simulink model "correlator_core"  (Simulink 7.1)
settings: Solver=ode45  StartTime=0.0  StopTime=10000  RelTol=1e-3
libraries: xbsIndex_r4 x658, cfa_library x168, casper_library_delays x4, casper_library_misc x2
(part 6 of 9)

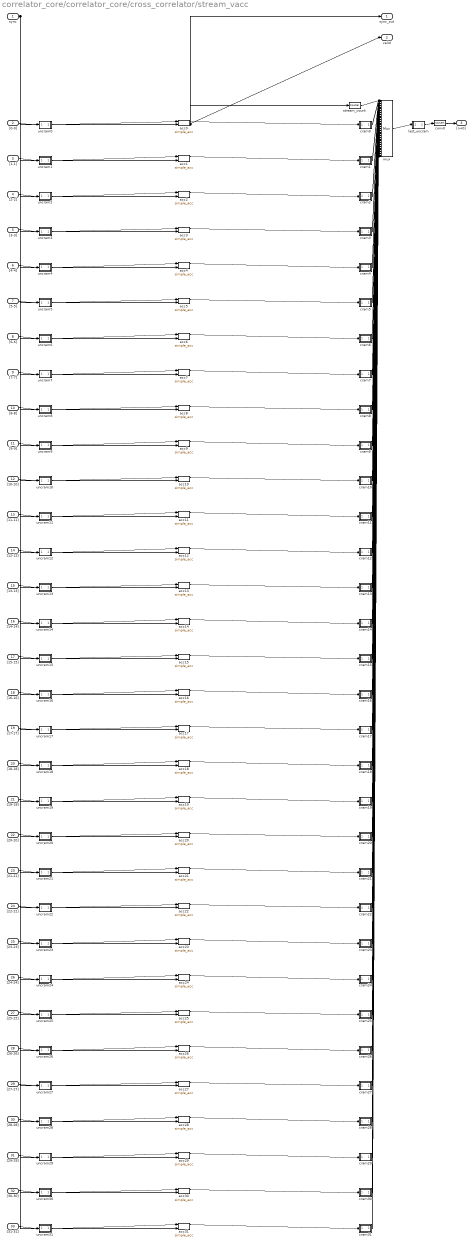
== system correlator_core/correlator_core/cross_correlator/stream_vacc ==
  sync : Inport
  "[0-0]" : Inport  Port=2
  "[1-1]" : Inport  Port=3
  "[2-2]" : Inport  Port=4
  "[3-3]" : Inport  Port=5
  "[4-4]" : Inport  Port=6
  "[5-5]" : Inport  Port=7
  "[6-6]" : Inport  Port=8
  "[7-7]" : Inport  Port=9
  "[8-8]" : Inport  Port=10
  "[9-9]" : Inport  Port=11
  "[10-10]" : Inport  Port=12
  "[11-11]" : Inport  Port=13
  "[12-12]" : Inport  Port=14
  "[13-13]" : Inport  Port=15
  "[14-14]" : Inport  Port=16
  "[15-15]" : Inport  Port=17
  "[16-16]" : Inport  Port=18
  "[17-17]" : Inport  Port=19
  "[18-18]" : Inport  Port=20
  "[19-19]" : Inport  Port=21
  "[20-20]" : Inport  Port=22
  "[21-21]" : Inport  Port=23
  "[22-22]" : Inport  Port=24
  "[23-23]" : Inport  Port=25
  "[24-24]" : Inport  Port=26
  "[25-25]" : Inport  Port=27
  "[26-26]" : Inport  Port=28
  "[27-27]" : Inport  Port=29
  "[28-28]" : Inport  Port=30
  "[29-29]" : Inport  Port=31
  "[30-30]" : Inport  Port=32
  "[31-31]" : Inport  Port=33
  acc0 : cfa_library/simple_acc  SystemSampleTime=-1  samples=5  bit_width=11  bin_pt=0  quantization=Truncate  overflow=Wrap  specify_add=off  add_spec=Fabric
      link override AddSub: quantization=Truncate  overflow=Wrap  use_behavioral_HDL=on  hw_selection=Fabric
  acc1 : cfa_library/simple_acc  SystemSampleTime=-1  samples=5  bit_width=11  bin_pt=0  quantization=Truncate  overflow=Wrap  specify_add=off  add_spec=Fabric
      link override AddSub: quantization=Truncate  overflow=Wrap  use_behavioral_HDL=on  hw_selection=Fabric
  acc10 : cfa_library/simple_acc  SystemSampleTime=-1  samples=5  bit_width=11  bin_pt=0  quantization=Truncate  overflow=Wrap  specify_add=off  add_spec=Fabric
      link override AddSub: quantization=Truncate  overflow=Wrap  use_behavioral_HDL=on  hw_selection=Fabric
  acc11 : cfa_library/simple_acc  SystemSampleTime=-1  samples=5  bit_width=11  bin_pt=0  quantization=Truncate  overflow=Wrap  specify_add=off  add_spec=Fabric
      link override AddSub: quantization=Truncate  overflow=Wrap  use_behavioral_HDL=on  hw_selection=Fabric
  acc12 : cfa_library/simple_acc  SystemSampleTime=-1  samples=5  bit_width=11  bin_pt=0  quantization=Truncate  overflow=Wrap  specify_add=off  add_spec=Fabric
      link override AddSub: quantization=Truncate  overflow=Wrap  use_behavioral_HDL=on  hw_selection=Fabric
  acc13 : cfa_library/simple_acc  SystemSampleTime=-1  samples=5  bit_width=11  bin_pt=0  quantization=Truncate  overflow=Wrap  specify_add=off  add_spec=Fabric
      link override AddSub: quantization=Truncate  overflow=Wrap  use_behavioral_HDL=on  hw_selection=Fabric
  acc14 : cfa_library/simple_acc  SystemSampleTime=-1  samples=5  bit_width=11  bin_pt=0  quantization=Truncate  overflow=Wrap  specify_add=off  add_spec=Fabric
      link override AddSub: quantization=Truncate  overflow=Wrap  use_behavioral_HDL=on  hw_selection=Fabric
  acc15 : cfa_library/simple_acc  SystemSampleTime=-1  samples=5  bit_width=11  bin_pt=0  quantization=Truncate  overflow=Wrap  specify_add=off  add_spec=Fabric
      link override AddSub: quantization=Truncate  overflow=Wrap  use_behavioral_HDL=on  hw_selection=Fabric
  acc16 : cfa_library/simple_acc  SystemSampleTime=-1  samples=5  bit_width=11  bin_pt=0  quantization=Truncate  overflow=Wrap  specify_add=off  add_spec=Fabric
      link override AddSub: quantization=Truncate  overflow=Wrap  use_behavioral_HDL=on  hw_selection=Fabric
  acc17 : cfa_library/simple_acc  SystemSampleTime=-1  samples=5  bit_width=11  bin_pt=0  quantization=Truncate  overflow=Wrap  specify_add=off  add_spec=Fabric
      link override AddSub: quantization=Truncate  overflow=Wrap  use_behavioral_HDL=on  hw_selection=Fabric
  acc18 : cfa_library/simple_acc  SystemSampleTime=-1  samples=5  bit_width=11  bin_pt=0  quantization=Truncate  overflow=Wrap  specify_add=off  add_spec=Fabric
      link override AddSub: quantization=Truncate  overflow=Wrap  use_behavioral_HDL=on  hw_selection=Fabric
  acc19 : cfa_library/simple_acc  SystemSampleTime=-1  samples=5  bit_width=11  bin_pt=0  quantization=Truncate  overflow=Wrap  specify_add=off  add_spec=Fabric
      link override AddSub: quantization=Truncate  overflow=Wrap  use_behavioral_HDL=on  hw_selection=Fabric
  acc2 : cfa_library/simple_acc  SystemSampleTime=-1  samples=5  bit_width=11  bin_pt=0  quantization=Truncate  overflow=Wrap  specify_add=off  add_spec=Fabric
      link override AddSub: quantization=Truncate  overflow=Wrap  use_behavioral_HDL=on  hw_selection=Fabric
  acc20 : cfa_library/simple_acc  SystemSampleTime=-1  samples=5  bit_width=11  bin_pt=0  quantization=Truncate  overflow=Wrap  specify_add=off  add_spec=Fabric
      link override AddSub: quantization=Truncate  overflow=Wrap  use_behavioral_HDL=on  hw_selection=Fabric
  acc21 : cfa_library/simple_acc  SystemSampleTime=-1  samples=5  bit_width=11  bin_pt=0  quantization=Truncate  overflow=Wrap  specify_add=off  add_spec=Fabric
      link override AddSub: quantization=Truncate  overflow=Wrap  use_behavioral_HDL=on  hw_selection=Fabric
  acc22 : cfa_library/simple_acc  SystemSampleTime=-1  samples=5  bit_width=11  bin_pt=0  quantization=Truncate  overflow=Wrap  specify_add=off  add_spec=Fabric
      link override AddSub: quantization=Truncate  overflow=Wrap  use_behavioral_HDL=on  hw_selection=Fabric
  acc23 : cfa_library/simple_acc  SystemSampleTime=-1  samples=5  bit_width=11  bin_pt=0  quantization=Truncate  overflow=Wrap  specify_add=off  add_spec=Fabric
      link override AddSub: quantization=Truncate  overflow=Wrap  use_behavioral_HDL=on  hw_selection=Fabric
  acc24 : cfa_library/simple_acc  SystemSampleTime=-1  samples=5  bit_width=11  bin_pt=0  quantization=Truncate  overflow=Wrap  specify_add=off  add_spec=Fabric
      link override AddSub: quantization=Truncate  overflow=Wrap  use_behavioral_HDL=on  hw_selection=Fabric
  acc25 : cfa_library/simple_acc  SystemSampleTime=-1  samples=5  bit_width=11  bin_pt=0  quantization=Truncate  overflow=Wrap  specify_add=off  add_spec=Fabric
      link override AddSub: quantization=Truncate  overflow=Wrap  use_behavioral_HDL=on  hw_selection=Fabric
  acc26 : cfa_library/simple_acc  SystemSampleTime=-1  samples=5  bit_width=11  bin_pt=0  quantization=Truncate  overflow=Wrap  specify_add=off  add_spec=Fabric
      link override AddSub: quantization=Truncate  overflow=Wrap  use_behavioral_HDL=on  hw_selection=Fabric
  acc27 : cfa_library/simple_acc  SystemSampleTime=-1  samples=5  bit_width=11  bin_pt=0  quantization=Truncate  overflow=Wrap  specify_add=off  add_spec=Fabric
      link override AddSub: quantization=Truncate  overflow=Wrap  use_behavioral_HDL=on  hw_selection=Fabric
  acc28 : cfa_library/simple_acc  SystemSampleTime=-1  samples=5  bit_width=11  bin_pt=0  quantization=Truncate  overflow=Wrap  specify_add=off  add_spec=Fabric
      link override AddSub: quantization=Truncate  overflow=Wrap  use_behavioral_HDL=on  hw_selection=Fabric
  acc29 : cfa_library/simple_acc  SystemSampleTime=-1  samples=5  bit_width=11  bin_pt=0  quantization=Truncate  overflow=Wrap  specify_add=off  add_spec=Fabric
      link override AddSub: quantization=Truncate  overflow=Wrap  use_behavioral_HDL=on  hw_selection=Fabric
  acc3 : cfa_library/simple_acc  SystemSampleTime=-1  samples=5  bit_width=11  bin_pt=0  quantization=Truncate  overflow=Wrap  specify_add=off  add_spec=Fabric
      link override AddSub: quantization=Truncate  overflow=Wrap  use_behavioral_HDL=on  hw_selection=Fabric
  acc30 : cfa_library/simple_acc  SystemSampleTime=-1  samples=5  bit_width=11  bin_pt=0  quantization=Truncate  overflow=Wrap  specify_add=off  add_spec=Fabric
      link override AddSub: quantization=Truncate  overflow=Wrap  use_behavioral_HDL=on  hw_selection=Fabric
  acc31 : cfa_library/simple_acc  SystemSampleTime=-1  samples=5  bit_width=11  bin_pt=0  quantization=Truncate  overflow=Wrap  specify_add=off  add_spec=Fabric
      link override AddSub: quantization=Truncate  overflow=Wrap  use_behavioral_HDL=on  hw_selection=Fabric
  acc4 : cfa_library/simple_acc  SystemSampleTime=-1  samples=5  bit_width=11  bin_pt=0  quantization=Truncate  overflow=Wrap  specify_add=off  add_spec=Fabric
      link override AddSub: quantization=Truncate  overflow=Wrap  use_behavioral_HDL=on  hw_selection=Fabric
  acc5 : cfa_library/simple_acc  SystemSampleTime=-1  samples=5  bit_width=11  bin_pt=0  quantization=Truncate  overflow=Wrap  specify_add=off  add_spec=Fabric
      link override AddSub: quantization=Truncate  overflow=Wrap  use_behavioral_HDL=on  hw_selection=Fabric
  acc6 : cfa_library/simple_acc  SystemSampleTime=-1  samples=5  bit_width=11  bin_pt=0  quantization=Truncate  overflow=Wrap  specify_add=off  add_spec=Fabric
      link override AddSub: quantization=Truncate  overflow=Wrap  use_behavioral_HDL=on  hw_selection=Fabric
  acc7 : cfa_library/simple_acc  SystemSampleTime=-1  samples=5  bit_width=11  bin_pt=0  quantization=Truncate  overflow=Wrap  specify_add=off  add_spec=Fabric
      link override AddSub: quantization=Truncate  overflow=Wrap  use_behavioral_HDL=on  hw_selection=Fabric
  acc8 : cfa_library/simple_acc  SystemSampleTime=-1  samples=5  bit_width=11  bin_pt=0  quantization=Truncate  overflow=Wrap  specify_add=off  add_spec=Fabric
      link override AddSub: quantization=Truncate  overflow=Wrap  use_behavioral_HDL=on  hw_selection=Fabric
  acc9 : cfa_library/simple_acc  SystemSampleTime=-1  samples=5  bit_width=11  bin_pt=0  quantization=Truncate  overflow=Wrap  specify_add=off  add_spec=Fabric
      link override AddSub: quantization=Truncate  overflow=Wrap  use_behavioral_HDL=on  hw_selection=Fabric
  conv0 : xbsIndex_r4/Convert  arith_type="Signed  (2's comp)"  n_bits=11  bin_pt=0  quantization=Truncate  overflow=Wrap  latency=0  dbl_ovrd=off  pipeline=off  block_type=convert
      settings: block_version=11.4
  cram0 : Subsystem  AncestorBlock=gavrt_library/cram  mask(cram){num_slice=1}
      mask prompts: num_slice "Number of slices"
      mask help: Concatenates inputs together after forcing binary point to zero.
      mask init:
      | cram_init(gcb, ...
      |     'num_slice', num_slice);
  cram1 : Subsystem  AncestorBlock=gavrt_library/cram  mask(cram){num_slice=1}
      mask prompts: num_slice "Number of slices"
      mask help: Concatenates inputs together after forcing binary point to zero.
      mask init:
      | cram_init(gcb, ...
      |     'num_slice', num_slice);
  cram10 : Subsystem  AncestorBlock=gavrt_library/cram  mask(cram){num_slice=1}
      mask prompts: num_slice "Number of slices"
      mask help: Concatenates inputs together after forcing binary point to zero.
      mask init:
      | cram_init(gcb, ...
      |     'num_slice', num_slice);
  cram11 : Subsystem  AncestorBlock=gavrt_library/cram  mask(cram){num_slice=1}
      mask prompts: num_slice "Number of slices"
      mask help: Concatenates inputs together after forcing binary point to zero.
      mask init:
      | cram_init(gcb, ...
      |     'num_slice', num_slice);
  cram12 : Subsystem  AncestorBlock=gavrt_library/cram  mask(cram){num_slice=1}
      mask prompts: num_slice "Number of slices"
      mask help: Concatenates inputs together after forcing binary point to zero.
      mask init:
      | cram_init(gcb, ...
      |     'num_slice', num_slice);
  cram13 : Subsystem  AncestorBlock=gavrt_library/cram  mask(cram){num_slice=1}
      mask prompts: num_slice "Number of slices"
      mask help: Concatenates inputs together after forcing binary point to zero.
      mask init:
      | cram_init(gcb, ...
      |     'num_slice', num_slice);
  cram14 : Subsystem  AncestorBlock=gavrt_library/cram  mask(cram){num_slice=1}
      mask prompts: num_slice "Number of slices"
      mask help: Concatenates inputs together after forcing binary point to zero.
      mask init:
      | cram_init(gcb, ...
      |     'num_slice', num_slice);
  cram15 : Subsystem  AncestorBlock=gavrt_library/cram  mask(cram){num_slice=1}
      mask prompts: num_slice "Number of slices"
      mask help: Concatenates inputs together after forcing binary point to zero.
      mask init:
      | cram_init(gcb, ...
      |     'num_slice', num_slice);
  cram16 : Subsystem  AncestorBlock=gavrt_library/cram  mask(cram){num_slice=1}
      mask prompts: num_slice "Number of slices"
      mask help: Concatenates inputs together after forcing binary point to zero.
      mask init:
      | cram_init(gcb, ...
      |     'num_slice', num_slice);
  cram17 : Subsystem  AncestorBlock=gavrt_library/cram  mask(cram){num_slice=1}
      mask prompts: num_slice "Number of slices"
      mask help: Concatenates inputs together after forcing binary point to zero.
      mask init:
      | cram_init(gcb, ...
      |     'num_slice', num_slice);
  cram18 : Subsystem  AncestorBlock=gavrt_library/cram  mask(cram){num_slice=1}
      mask prompts: num_slice "Number of slices"
      mask help: Concatenates inputs together after forcing binary point to zero.
      mask init:
      | cram_init(gcb, ...
      |     'num_slice', num_slice);
  cram19 : Subsystem  AncestorBlock=gavrt_library/cram  mask(cram){num_slice=1}
      mask prompts: num_slice "Number of slices"
      mask help: Concatenates inputs together after forcing binary point to zero.
      mask init:
      | cram_init(gcb, ...
      |     'num_slice', num_slice);
  cram2 : Subsystem  AncestorBlock=gavrt_library/cram  mask(cram){num_slice=1}
      mask prompts: num_slice "Number of slices"
      mask help: Concatenates inputs together after forcing binary point to zero.
      mask init:
      | cram_init(gcb, ...
      |     'num_slice', num_slice);
  cram20 : Subsystem  AncestorBlock=gavrt_library/cram  mask(cram){num_slice=1}
      mask prompts: num_slice "Number of slices"
      mask help: Concatenates inputs together after forcing binary point to zero.
      mask init:
      | cram_init(gcb, ...
      |     'num_slice', num_slice);
  cram21 : Subsystem  AncestorBlock=gavrt_library/cram  mask(cram){num_slice=1}
      mask prompts: num_slice "Number of slices"
      mask help: Concatenates inputs together after forcing binary point to zero.
      mask init:
      | cram_init(gcb, ...
      |     'num_slice', num_slice);
  cram22 : Subsystem  AncestorBlock=gavrt_library/cram  mask(cram){num_slice=1}
      mask prompts: num_slice "Number of slices"
      mask help: Concatenates inputs together after forcing binary point to zero.
      mask init:
      | cram_init(gcb, ...
      |     'num_slice', num_slice);
  cram23 : Subsystem  AncestorBlock=gavrt_library/cram  mask(cram){num_slice=1}
      mask prompts: num_slice "Number of slices"
      mask help: Concatenates inputs together after forcing binary point to zero.
      mask init:
      | cram_init(gcb, ...
      |     'num_slice', num_slice);
  cram24 : Subsystem  AncestorBlock=gavrt_library/cram  mask(cram){num_slice=1}
      mask prompts: num_slice "Number of slices"
      mask help: Concatenates inputs together after forcing binary point to zero.
      mask init:
      | cram_init(gcb, ...
      |     'num_slice', num_slice);
  cram25 : Subsystem  AncestorBlock=gavrt_library/cram  mask(cram){num_slice=1}
      mask prompts: num_slice "Number of slices"
      mask help: Concatenates inputs together after forcing binary point to zero.
      mask init:
      | cram_init(gcb, ...
      |     'num_slice', num_slice);
  cram26 : Subsystem  AncestorBlock=gavrt_library/cram  mask(cram){num_slice=1}
      mask prompts: num_slice "Number of slices"
      mask help: Concatenates inputs together after forcing binary point to zero.
      mask init:
      | cram_init(gcb, ...
      |     'num_slice', num_slice);
  cram27 : Subsystem  AncestorBlock=gavrt_library/cram  mask(cram){num_slice=1}
      mask prompts: num_slice "Number of slices"
      mask help: Concatenates inputs together after forcing binary point to zero.
      mask init:
      | cram_init(gcb, ...
      |     'num_slice', num_slice);
  cram28 : Subsystem  AncestorBlock=gavrt_library/cram  mask(cram){num_slice=1}
      mask prompts: num_slice "Number of slices"
      mask help: Concatenates inputs together after forcing binary point to zero.
      mask init:
      | cram_init(gcb, ...
      |     'num_slice', num_slice);
  cram29 : Subsystem  AncestorBlock=gavrt_library/cram  mask(cram){num_slice=1}
      mask prompts: num_slice "Number of slices"
      mask help: Concatenates inputs together after forcing binary point to zero.
      mask init:
      | cram_init(gcb, ...
      |     'num_slice', num_slice);
  cram3 : Subsystem  AncestorBlock=gavrt_library/cram  mask(cram){num_slice=1}
      mask prompts: num_slice "Number of slices"
      mask help: Concatenates inputs together after forcing binary point to zero.
      mask init:
      | cram_init(gcb, ...
      |     'num_slice', num_slice);
  cram30 : Subsystem  AncestorBlock=gavrt_library/cram  mask(cram){num_slice=1}
      mask prompts: num_slice "Number of slices"
      mask help: Concatenates inputs together after forcing binary point to zero.
      mask init:
      | cram_init(gcb, ...
      |     'num_slice', num_slice);
  cram31 : Subsystem  AncestorBlock=gavrt_library/cram  mask(cram){num_slice=1}
      mask prompts: num_slice "Number of slices"
      mask help: Concatenates inputs together after forcing binary point to zero.
      mask init:
      | cram_init(gcb, ...
      |     'num_slice', num_slice);
  cram4 : Subsystem  AncestorBlock=gavrt_library/cram  mask(cram){num_slice=1}
      mask prompts: num_slice "Number of slices"
      mask help: Concatenates inputs together after forcing binary point to zero.
      mask init:
      | cram_init(gcb, ...
      |     'num_slice', num_slice);
  cram5 : Subsystem  AncestorBlock=gavrt_library/cram  mask(cram){num_slice=1}
      mask prompts: num_slice "Number of slices"
      mask help: Concatenates inputs together after forcing binary point to zero.
      mask init:
      | cram_init(gcb, ...
      |     'num_slice', num_slice);
  cram6 : Subsystem  AncestorBlock=gavrt_library/cram  mask(cram){num_slice=1}
      mask prompts: num_slice "Number of slices"
      mask help: Concatenates inputs together after forcing binary point to zero.
      mask init:
      | cram_init(gcb, ...
      |     'num_slice', num_slice);
  cram7 : Subsystem  AncestorBlock=gavrt_library/cram  mask(cram){num_slice=1}
      mask prompts: num_slice "Number of slices"
      mask help: Concatenates inputs together after forcing binary point to zero.
      mask init:
      | cram_init(gcb, ...
      |     'num_slice', num_slice);
  cram8 : Subsystem  AncestorBlock=gavrt_library/cram  mask(cram){num_slice=1}
      mask prompts: num_slice "Number of slices"
      mask help: Concatenates inputs together after forcing binary point to zero.
      mask init:
      | cram_init(gcb, ...
      |     'num_slice', num_slice);
  cram9 : Subsystem  AncestorBlock=gavrt_library/cram  mask(cram){num_slice=1}
      mask prompts: num_slice "Number of slices"
      mask help: Concatenates inputs together after forcing binary point to zero.
      mask init:
      | cram_init(gcb, ...
      |     'num_slice', num_slice);
  last_uncram : Subsystem  AncestorBlock=gavrt_library/uncram  mask(uncram){num_slice=1, slice_width=11, bin_pt=0, arith_type=1}
      mask prompts: num_slice "Number of slices"; slice_width "Slice Width"; bin_pt "Output Binary Point"; arith_type "Output Arithmetic Type (0=Unsigned, 1=Signed)"
      mask help: Takes a concatenated input and slices it up into even pieces and reinterprets them as signed fixed point numbers with a given binary point.
      mask init:
      | uncram_init(gcb, ...
      |     'num_slice', num_slice, ...
      |     'slice_width', slice_width, ...
      |     'bin_pt', bin_pt, ...
      |     'arith_type', arith_type);
      settings: AttributesFormatString=Fix_11_0
  mux : xbsIndex_r4/Mux  inputs=32  en=off  latency=0  precision=Full  arith_type=Unsigned  n_bits=16  bin_pt=14  quantization=Truncate  overflow=Wrap  dbl_ovrd=off  block_type=mux
      settings: block_version=11.4
  stream_count : xbsIndex_r4/Counter  cnt_type=Free Running  cnt_to=Inf  operation=Up  start_count=0  cnt_by_val=1  arith_type=Unsigned  n_bits=5  bin_pt=0  load_pin=off  rst=on  en=off  explicit_period=on  period=1  dbl_ovrd=off  use_behavioral_HDL=off  use_rpm=off  implementation=Fabric  block_type=counter
      settings: block_version=11.4
  uncram0 : Subsystem  AncestorBlock=gavrt_library/uncram  mask(uncram){num_slice=1, slice_width=7, bin_pt=0, arith_type=1}
      mask prompts: num_slice "Number of slices"; slice_width "Slice Width"; bin_pt "Output Binary Point"; arith_type "Output Arithmetic Type (0=Unsigned, 1=Signed)"
      mask help: Takes a concatenated input and slices it up into even pieces and reinterprets them as signed fixed point numbers with a given binary point.
      mask init:
      | uncram_init(gcb, ...
      |     'num_slice', num_slice, ...
      |     'slice_width', slice_width, ...
      |     'bin_pt', bin_pt, ...
      |     'arith_type', arith_type);
      settings: AttributesFormatString=Fix_7_0
  uncram1 : Subsystem  AncestorBlock=gavrt_library/uncram  mask(uncram){num_slice=1, slice_width=7, bin_pt=0, arith_type=1}
      mask prompts: num_slice "Number of slices"; slice_width "Slice Width"; bin_pt "Output Binary Point"; arith_type "Output Arithmetic Type (0=Unsigned, 1=Signed)"
      mask help: Takes a concatenated input and slices it up into even pieces and reinterprets them as signed fixed point numbers with a given binary point.
      mask init:
      | uncram_init(gcb, ...
      |     'num_slice', num_slice, ...
      |     'slice_width', slice_width, ...
      |     'bin_pt', bin_pt, ...
      |     'arith_type', arith_type);
      settings: AttributesFormatString=Fix_7_0
  uncram10 : Subsystem  AncestorBlock=gavrt_library/uncram  mask(uncram){num_slice=1, slice_width=7, bin_pt=0, arith_type=1}
      mask prompts: num_slice "Number of slices"; slice_width "Slice Width"; bin_pt "Output Binary Point"; arith_type "Output Arithmetic Type (0=Unsigned, 1=Signed)"
      mask help: Takes a concatenated input and slices it up into even pieces and reinterprets them as signed fixed point numbers with a given binary point.
      mask init:
      | uncram_init(gcb, ...
      |     'num_slice', num_slice, ...
      |     'slice_width', slice_width, ...
      |     'bin_pt', bin_pt, ...
      |     'arith_type', arith_type);
      settings: AttributesFormatString=Fix_7_0
  uncram11 : Subsystem  AncestorBlock=gavrt_library/uncram  mask(uncram){num_slice=1, slice_width=7, bin_pt=0, arith_type=1}
      mask prompts: num_slice "Number of slices"; slice_width "Slice Width"; bin_pt "Output Binary Point"; arith_type "Output Arithmetic Type (0=Unsigned, 1=Signed)"
      mask help: Takes a concatenated input and slices it up into even pieces and reinterprets them as signed fixed point numbers with a given binary point.
      mask init:
      | uncram_init(gcb, ...
      |     'num_slice', num_slice, ...
      |     'slice_width', slice_width, ...
      |     'bin_pt', bin_pt, ...
      |     'arith_type', arith_type);
      settings: AttributesFormatString=Fix_7_0
  uncram12 : Subsystem  AncestorBlock=gavrt_library/uncram  mask(uncram){num_slice=1, slice_width=7, bin_pt=0, arith_type=1}
      mask prompts: num_slice "Number of slices"; slice_width "Slice Width"; bin_pt "Output Binary Point"; arith_type "Output Arithmetic Type (0=Unsigned, 1=Signed)"
      mask help: Takes a concatenated input and slices it up into even pieces and reinterprets them as signed fixed point numbers with a given binary point.
      mask init:
      | uncram_init(gcb, ...
      |     'num_slice', num_slice, ...
      |     'slice_width', slice_width, ...
      |     'bin_pt', bin_pt, ...
      |     'arith_type', arith_type);
      settings: AttributesFormatString=Fix_7_0
  uncram13 : Subsystem  AncestorBlock=gavrt_library/uncram  mask(uncram){num_slice=1, slice_width=7, bin_pt=0, arith_type=1}
      mask prompts: num_slice "Number of slices"; slice_width "Slice Width"; bin_pt "Output Binary Point"; arith_type "Output Arithmetic Type (0=Unsigned, 1=Signed)"
      mask help: Takes a concatenated input and slices it up into even pieces and reinterprets them as signed fixed point numbers with a given binary point.
      mask init:
      | uncram_init(gcb, ...
      |     'num_slice', num_slice, ...
      |     'slice_width', slice_width, ...
      |     'bin_pt', bin_pt, ...
      |     'arith_type', arith_type);
      settings: AttributesFormatString=Fix_7_0
  uncram14 : Subsystem  AncestorBlock=gavrt_library/uncram  mask(uncram){num_slice=1, slice_width=7, bin_pt=0, arith_type=1}
      mask prompts: num_slice "Number of slices"; slice_width "Slice Width"; bin_pt "Output Binary Point"; arith_type "Output Arithmetic Type (0=Unsigned, 1=Signed)"
      mask help: Takes a concatenated input and slices it up into even pieces and reinterprets them as signed fixed point numbers with a given binary point.
      mask init:
      | uncram_init(gcb, ...
      |     'num_slice', num_slice, ...
      |     'slice_width', slice_width, ...
      |     'bin_pt', bin_pt, ...
      |     'arith_type', arith_type);
      settings: AttributesFormatString=Fix_7_0
  uncram15 : Subsystem  AncestorBlock=gavrt_library/uncram  mask(uncram){num_slice=1, slice_width=7, bin_pt=0, arith_type=1}
      mask prompts: num_slice "Number of slices"; slice_width "Slice Width"; bin_pt "Output Binary Point"; arith_type "Output Arithmetic Type (0=Unsigned, 1=Signed)"
      mask help: Takes a concatenated input and slices it up into even pieces and reinterprets them as signed fixed point numbers with a given binary point.
      mask init:
      | uncram_init(gcb, ...
      |     'num_slice', num_slice, ...
      |     'slice_width', slice_width, ...
      |     'bin_pt', bin_pt, ...
      |     'arith_type', arith_type);
      settings: AttributesFormatString=Fix_7_0
  uncram16 : Subsystem  AncestorBlock=gavrt_library/uncram  mask(uncram){num_slice=1, slice_width=7, bin_pt=0, arith_type=1}
      mask prompts: num_slice "Number of slices"; slice_width "Slice Width"; bin_pt "Output Binary Point"; arith_type "Output Arithmetic Type (0=Unsigned, 1=Signed)"
      mask help: Takes a concatenated input and slices it up into even pieces and reinterprets them as signed fixed point numbers with a given binary point.
      mask init:
      | uncram_init(gcb, ...
      |     'num_slice', num_slice, ...
      |     'slice_width', slice_width, ...
      |     'bin_pt', bin_pt, ...
      |     'arith_type', arith_type);
      settings: AttributesFormatString=Fix_7_0
  uncram17 : Subsystem  AncestorBlock=gavrt_library/uncram  mask(uncram){num_slice=1, slice_width=7, bin_pt=0, arith_type=1}
      mask prompts: num_slice "Number of slices"; slice_width "Slice Width"; bin_pt "Output Binary Point"; arith_type "Output Arithmetic Type (0=Unsigned, 1=Signed)"
      mask help: Takes a concatenated input and slices it up into even pieces and reinterprets them as signed fixed point numbers with a given binary point.
      mask init:
      | uncram_init(gcb, ...
      |     'num_slice', num_slice, ...
      |     'slice_width', slice_width, ...
      |     'bin_pt', bin_pt, ...
      |     'arith_type', arith_type);
      settings: AttributesFormatString=Fix_7_0
  uncram18 : Subsystem  AncestorBlock=gavrt_library/uncram  mask(uncram){num_slice=1, slice_width=7, bin_pt=0, arith_type=1}
      mask prompts: num_slice "Number of slices"; slice_width "Slice Width"; bin_pt "Output Binary Point"; arith_type "Output Arithmetic Type (0=Unsigned, 1=Signed)"
      mask help: Takes a concatenated input and slices it up into even pieces and reinterprets them as signed fixed point numbers with a given binary point.
      mask init:
      | uncram_init(gcb, ...
      |     'num_slice', num_slice, ...
      |     'slice_width', slice_width, ...
      |     'bin_pt', bin_pt, ...
      |     'arith_type', arith_type);
      settings: AttributesFormatString=Fix_7_0
  uncram19 : Subsystem  AncestorBlock=gavrt_library/uncram  mask(uncram){num_slice=1, slice_width=7, bin_pt=0, arith_type=1}
      mask prompts: num_slice "Number of slices"; slice_width "Slice Width"; bin_pt "Output Binary Point"; arith_type "Output Arithmetic Type (0=Unsigned, 1=Signed)"
      mask help: Takes a concatenated input and slices it up into even pieces and reinterprets them as signed fixed point numbers with a given binary point.
      mask init:
      | uncram_init(gcb, ...
      |     'num_slice', num_slice, ...
      |     'slice_width', slice_width, ...
      |     'bin_pt', bin_pt, ...
      |     'arith_type', arith_type);
      settings: AttributesFormatString=Fix_7_0
  uncram2 : Subsystem  AncestorBlock=gavrt_library/uncram  mask(uncram){num_slice=1, slice_width=7, bin_pt=0, arith_type=1}
      mask prompts: num_slice "Number of slices"; slice_width "Slice Width"; bin_pt "Output Binary Point"; arith_type "Output Arithmetic Type (0=Unsigned, 1=Signed)"
      mask help: Takes a concatenated input and slices it up into even pieces and reinterprets them as signed fixed point numbers with a given binary point.
      mask init:
      | uncram_init(gcb, ...
      |     'num_slice', num_slice, ...
      |     'slice_width', slice_width, ...
      |     'bin_pt', bin_pt, ...
      |     'arith_type', arith_type);
      settings: AttributesFormatString=Fix_7_0
  uncram20 : Subsystem  AncestorBlock=gavrt_library/uncram  mask(uncram){num_slice=1, slice_width=7, bin_pt=0, arith_type=1}
      mask prompts: num_slice "Number of slices"; slice_width "Slice Width"; bin_pt "Output Binary Point"; arith_type "Output Arithmetic Type (0=Unsigned, 1=Signed)"
      mask help: Takes a concatenated input and slices it up into even pieces and reinterprets them as signed fixed point numbers with a given binary point.
      mask init:
      | uncram_init(gcb, ...
      |     'num_slice', num_slice, ...
      |     'slice_width', slice_width, ...
      |     'bin_pt', bin_pt, ...
      |     'arith_type', arith_type);
      settings: AttributesFormatString=Fix_7_0
  uncram21 : Subsystem  AncestorBlock=gavrt_library/uncram  mask(uncram){num_slice=1, slice_width=7, bin_pt=0, arith_type=1}
      mask prompts: num_slice "Number of slices"; slice_width "Slice Width"; bin_pt "Output Binary Point"; arith_type "Output Arithmetic Type (0=Unsigned, 1=Signed)"
      mask help: Takes a concatenated input and slices it up into even pieces and reinterprets them as signed fixed point numbers with a given binary point.
      mask init:
      | uncram_init(gcb, ...
      |     'num_slice', num_slice, ...
      |     'slice_width', slice_width, ...
      |     'bin_pt', bin_pt, ...
      |     'arith_type', arith_type);
      settings: AttributesFormatString=Fix_7_0
  uncram22 : Subsystem  AncestorBlock=gavrt_library/uncram  mask(uncram){num_slice=1, slice_width=7, bin_pt=0, arith_type=1}
      mask prompts: num_slice "Number of slices"; slice_width "Slice Width"; bin_pt "Output Binary Point"; arith_type "Output Arithmetic Type (0=Unsigned, 1=Signed)"
      mask help: Takes a concatenated input and slices it up into even pieces and reinterprets them as signed fixed point numbers with a given binary point.
      mask init:
      | uncram_init(gcb, ...
      |     'num_slice', num_slice, ...
      |     'slice_width', slice_width, ...
      |     'bin_pt', bin_pt, ...
      |     'arith_type', arith_type);
      settings: AttributesFormatString=Fix_7_0
  uncram23 : Subsystem  AncestorBlock=gavrt_library/uncram  mask(uncram){num_slice=1, slice_width=7, bin_pt=0, arith_type=1}
      mask prompts: num_slice "Number of slices"; slice_width "Slice Width"; bin_pt "Output Binary Point"; arith_type "Output Arithmetic Type (0=Unsigned, 1=Signed)"
      mask help: Takes a concatenated input and slices it up into even pieces and reinterprets them as signed fixed point numbers with a given binary point.
      mask init:
      | uncram_init(gcb, ...
      |     'num_slice', num_slice, ...
      |     'slice_width', slice_width, ...
      |     'bin_pt', bin_pt, ...
      |     'arith_type', arith_type);
      settings: AttributesFormatString=Fix_7_0
  uncram24 : Subsystem  AncestorBlock=gavrt_library/uncram  mask(uncram){num_slice=1, slice_width=7, bin_pt=0, arith_type=1}
      mask prompts: num_slice "Number of slices"; slice_width "Slice Width"; bin_pt "Output Binary Point"; arith_type "Output Arithmetic Type (0=Unsigned, 1=Signed)"
      mask help: Takes a concatenated input and slices it up into even pieces and reinterprets them as signed fixed point numbers with a given binary point.
      mask init:
      | uncram_init(gcb, ...
      |     'num_slice', num_slice, ...
      |     'slice_width', slice_width, ...
      |     'bin_pt', bin_pt, ...
      |     'arith_type', arith_type);
      settings: AttributesFormatString=Fix_7_0
  uncram25 : Subsystem  AncestorBlock=gavrt_library/uncram  mask(uncram){num_slice=1, slice_width=7, bin_pt=0, arith_type=1}
      mask prompts: num_slice "Number of slices"; slice_width "Slice Width"; bin_pt "Output Binary Point"; arith_type "Output Arithmetic Type (0=Unsigned, 1=Signed)"
      mask help: Takes a concatenated input and slices it up into even pieces and reinterprets them as signed fixed point numbers with a given binary point.
      mask init:
      | uncram_init(gcb, ...
      |     'num_slice', num_slice, ...
      |     'slice_width', slice_width, ...
      |     'bin_pt', bin_pt, ...
      |     'arith_type', arith_type);
      settings: AttributesFormatString=Fix_7_0
  uncram26 : Subsystem  AncestorBlock=gavrt_library/uncram  mask(uncram){num_slice=1, slice_width=7, bin_pt=0, arith_type=1}
      mask prompts: num_slice "Number of slices"; slice_width "Slice Width"; bin_pt "Output Binary Point"; arith_type "Output Arithmetic Type (0=Unsigned, 1=Signed)"
      mask help: Takes a concatenated input and slices it up into even pieces and reinterprets them as signed fixed point numbers with a given binary point.
      mask init:
      | uncram_init(gcb, ...
      |     'num_slice', num_slice, ...
      |     'slice_width', slice_width, ...
      |     'bin_pt', bin_pt, ...
      |     'arith_type', arith_type);
      settings: AttributesFormatString=Fix_7_0
  uncram27 : Subsystem  AncestorBlock=gavrt_library/uncram  mask(uncram){num_slice=1, slice_width=7, bin_pt=0, arith_type=1}
      mask prompts: num_slice "Number of slices"; slice_width "Slice Width"; bin_pt "Output Binary Point"; arith_type "Output Arithmetic Type (0=Unsigned, 1=Signed)"
      mask help: Takes a concatenated input and slices it up into even pieces and reinterprets them as signed fixed point numbers with a given binary point.
      mask init:
      | uncram_init(gcb, ...
      |     'num_slice', num_slice, ...
      |     'slice_width', slice_width, ...
      |     'bin_pt', bin_pt, ...
      |     'arith_type', arith_type);
      settings: AttributesFormatString=Fix_7_0
  uncram28 : Subsystem  AncestorBlock=gavrt_library/uncram  mask(uncram){num_slice=1, slice_width=7, bin_pt=0, arith_type=1}
      mask prompts: num_slice "Number of slices"; slice_width "Slice Width"; bin_pt "Output Binary Point"; arith_type "Output Arithmetic Type (0=Unsigned, 1=Signed)"
      mask help: Takes a concatenated input and slices it up into even pieces and reinterprets them as signed fixed point numbers with a given binary point.
      mask init:
      | uncram_init(gcb, ...
      |     'num_slice', num_slice, ...
      |     'slice_width', slice_width, ...
      |     'bin_pt', bin_pt, ...
      |     'arith_type', arith_type);
      settings: AttributesFormatString=Fix_7_0
  uncram29 : Subsystem  AncestorBlock=gavrt_library/uncram  mask(uncram){num_slice=1, slice_width=7, bin_pt=0, arith_type=1}
      mask prompts: num_slice "Number of slices"; slice_width "Slice Width"; bin_pt "Output Binary Point"; arith_type "Output Arithmetic Type (0=Unsigned, 1=Signed)"
      mask help: Takes a concatenated input and slices it up into even pieces and reinterprets them as signed fixed point numbers with a given binary point.
      mask init:
      | uncram_init(gcb, ...
      |     'num_slice', num_slice, ...
      |     'slice_width', slice_width, ...
      |     'bin_pt', bin_pt, ...
      |     'arith_type', arith_type);
      settings: AttributesFormatString=Fix_7_0
  uncram3 : Subsystem  AncestorBlock=gavrt_library/uncram  mask(uncram){num_slice=1, slice_width=7, bin_pt=0, arith_type=1}
      mask prompts: num_slice "Number of slices"; slice_width "Slice Width"; bin_pt "Output Binary Point"; arith_type "Output Arithmetic Type (0=Unsigned, 1=Signed)"
      mask help: Takes a concatenated input and slices it up into even pieces and reinterprets them as signed fixed point numbers with a given binary point.
      mask init:
      | uncram_init(gcb, ...
      |     'num_slice', num_slice, ...
      |     'slice_width', slice_width, ...
      |     'bin_pt', bin_pt, ...
      |     'arith_type', arith_type);
      settings: AttributesFormatString=Fix_7_0
  uncram30 : Subsystem  AncestorBlock=gavrt_library/uncram  mask(uncram){num_slice=1, slice_width=7, bin_pt=0, arith_type=1}
      mask prompts: num_slice "Number of slices"; slice_width "Slice Width"; bin_pt "Output Binary Point"; arith_type "Output Arithmetic Type (0=Unsigned, 1=Signed)"
      mask help: Takes a concatenated input and slices it up into even pieces and reinterprets them as signed fixed point numbers with a given binary point.
      mask init:
      | uncram_init(gcb, ...
      |     'num_slice', num_slice, ...
      |     'slice_width', slice_width, ...
      |     'bin_pt', bin_pt, ...
      |     'arith_type', arith_type);
      settings: AttributesFormatString=Fix_7_0
  uncram31 : Subsystem  AncestorBlock=gavrt_library/uncram  mask(uncram){num_slice=1, slice_width=7, bin_pt=0, arith_type=1}
      mask prompts: num_slice "Number of slices"; slice_width "Slice Width"; bin_pt "Output Binary Point"; arith_type "Output Arithmetic Type (0=Unsigned, 1=Signed)"
      mask help: Takes a concatenated input and slices it up into even pieces and reinterprets them as signed fixed point numbers with a given binary point.
      mask init:
      | uncram_init(gcb, ...
      |     'num_slice', num_slice, ...
      |     'slice_width', slice_width, ...
      |     'bin_pt', bin_pt, ...
      |     'arith_type', arith_type);
      settings: AttributesFormatString=Fix_7_0
  uncram4 : Subsystem  AncestorBlock=gavrt_library/uncram  mask(uncram){num_slice=1, slice_width=7, bin_pt=0, arith_type=1}
      mask prompts: num_slice "Number of slices"; slice_width "Slice Width"; bin_pt "Output Binary Point"; arith_type "Output Arithmetic Type (0=Unsigned, 1=Signed)"
      mask help: Takes a concatenated input and slices it up into even pieces and reinterprets them as signed fixed point numbers with a given binary point.
      mask init:
      | uncram_init(gcb, ...
      |     'num_slice', num_slice, ...
      |     'slice_width', slice_width, ...
      |     'bin_pt', bin_pt, ...
      |     'arith_type', arith_type);
      settings: AttributesFormatString=Fix_7_0
  uncram5 : Subsystem  AncestorBlock=gavrt_library/uncram  mask(uncram){num_slice=1, slice_width=7, bin_pt=0, arith_type=1}
      mask prompts: num_slice "Number of slices"; slice_width "Slice Width"; bin_pt "Output Binary Point"; arith_type "Output Arithmetic Type (0=Unsigned, 1=Signed)"
      mask help: Takes a concatenated input and slices it up into even pieces and reinterprets them as signed fixed point numbers with a given binary point.
      mask init:
      | uncram_init(gcb, ...
      |     'num_slice', num_slice, ...
      |     'slice_width', slice_width, ...
      |     'bin_pt', bin_pt, ...
      |     'arith_type', arith_type);
      settings: AttributesFormatString=Fix_7_0
  uncram6 : Subsystem  AncestorBlock=gavrt_library/uncram  mask(uncram){num_slice=1, slice_width=7, bin_pt=0, arith_type=1}
      mask prompts: num_slice "Number of slices"; slice_width "Slice Width"; bin_pt "Output Binary Point"; arith_type "Output Arithmetic Type (0=Unsigned, 1=Signed)"
      mask help: Takes a concatenated input and slices it up into even pieces and reinterprets them as signed fixed point numbers with a given binary point.
      mask init:
      | uncram_init(gcb, ...
      |     'num_slice', num_slice, ...
      |     'slice_width', slice_width, ...
      |     'bin_pt', bin_pt, ...
      |     'arith_type', arith_type);
      settings: AttributesFormatString=Fix_7_0
  uncram7 : Subsystem  AncestorBlock=gavrt_library/uncram  mask(uncram){num_slice=1, slice_width=7, bin_pt=0, arith_type=1}
      mask prompts: num_slice "Number of slices"; slice_width "Slice Width"; bin_pt "Output Binary Point"; arith_type "Output Arithmetic Type (0=Unsigned, 1=Signed)"
      mask help: Takes a concatenated input and slices it up into even pieces and reinterprets them as signed fixed point numbers with a given binary point.
      mask init:
      | uncram_init(gcb, ...
      |     'num_slice', num_slice, ...
      |     'slice_width', slice_width, ...
      |     'bin_pt', bin_pt, ...
      |     'arith_type', arith_type);
      settings: AttributesFormatString=Fix_7_0
  uncram8 : Subsystem  AncestorBlock=gavrt_library/uncram  mask(uncram){num_slice=1, slice_width=7, bin_pt=0, arith_type=1}
      mask prompts: num_slice "Number of slices"; slice_width "Slice Width"; bin_pt "Output Binary Point"; arith_type "Output Arithmetic Type (0=Unsigned, 1=Signed)"
      mask help: Takes a concatenated input and slices it up into even pieces and reinterprets them as signed fixed point numbers with a given binary point.
      mask init:
      | uncram_init(gcb, ...
      |     'num_slice', num_slice, ...
      |     'slice_width', slice_width, ...
      |     'bin_pt', bin_pt, ...
      |     'arith_type', arith_type);
      settings: AttributesFormatString=Fix_7_0
  uncram9 : Subsystem  AncestorBlock=gavrt_library/uncram  mask(uncram){num_slice=1, slice_width=7, bin_pt=0, arith_type=1}
      mask prompts: num_slice "Number of slices"; slice_width "Slice Width"; bin_pt "Output Binary Point"; arith_type "Output Arithmetic Type (0=Unsigned, 1=Signed)"
      mask help: Takes a concatenated input and slices it up into even pieces and reinterprets them as signed fixed point numbers with a given binary point.
      mask init:
      | uncram_init(gcb, ...
      |     'num_slice', num_slice, ...
      |     'slice_width', slice_width, ...
      |     'bin_pt', bin_pt, ...
      |     'arith_type', arith_type);
      settings: AttributesFormatString=Fix_7_0
  sync_out : Outport
  valid : Outport  Port=2
  "[n+0]" : Outport  Port=3
  wires:
  "[0-0]"/1 -> uncram0/1(In)
  uncram0/1(Out1) -> acc0/1
  sync/1 -> acc0/2, acc1/2, acc2/2, acc3/2, acc4/2, acc5/2, acc6/2, acc7/2, acc8/2, acc9/2, acc10/2, acc11/2, acc12/2, acc13/2, acc14/2, acc15/2, acc16/2, acc17/2, acc18/2, acc19/2, acc20/2, acc21/2, acc22/2, acc23/2, acc24/2, acc25/2, acc26/2, acc27/2, acc28/2, acc29/2, acc30/2, acc31/2
  acc0/1 -> cram0/1(In1)
  "[1-1]"/1 -> uncram1/1(In)
  uncram1/1(Out1) -> acc1/1
  acc1/1 -> cram1/1(In1)
  "[2-2]"/1 -> uncram2/1(In)
  uncram2/1(Out1) -> acc2/1
  acc2/1 -> cram2/1(In1)
  "[3-3]"/1 -> uncram3/1(In)
  uncram3/1(Out1) -> acc3/1
  acc3/1 -> cram3/1(In1)
  "[4-4]"/1 -> uncram4/1(In)
  uncram4/1(Out1) -> acc4/1
  acc4/1 -> cram4/1(In1)
  "[5-5]"/1 -> uncram5/1(In)
  uncram5/1(Out1) -> acc5/1
  acc5/1 -> cram5/1(In1)
  "[6-6]"/1 -> uncram6/1(In)
  uncram6/1(Out1) -> acc6/1
  acc6/1 -> cram6/1(In1)
  "[7-7]"/1 -> uncram7/1(In)
  uncram7/1(Out1) -> acc7/1
  acc7/1 -> cram7/1(In1)
  "[8-8]"/1 -> uncram8/1(In)
  uncram8/1(Out1) -> acc8/1
  acc8/1 -> cram8/1(In1)
  "[9-9]"/1 -> uncram9/1(In)
  uncram9/1(Out1) -> acc9/1
  acc9/1 -> cram9/1(In1)
  "[10-10]"/1 -> uncram10/1(In)
  uncram10/1(Out1) -> acc10/1
  acc10/1 -> cram10/1(In1)
  "[11-11]"/1 -> uncram11/1(In)
  uncram11/1(Out1) -> acc11/1
  acc11/1 -> cram11/1(In1)
  "[12-12]"/1 -> uncram12/1(In)
  uncram12/1(Out1) -> acc12/1
  acc12/1 -> cram12/1(In1)
  "[13-13]"/1 -> uncram13/1(In)
  uncram13/1(Out1) -> acc13/1
  acc13/1 -> cram13/1(In1)
  "[14-14]"/1 -> uncram14/1(In)
  uncram14/1(Out1) -> acc14/1
  acc14/1 -> cram14/1(In1)
  "[15-15]"/1 -> uncram15/1(In)
  uncram15/1(Out1) -> acc15/1
  acc15/1 -> cram15/1(In1)
  "[16-16]"/1 -> uncram16/1(In)
  uncram16/1(Out1) -> acc16/1
  acc16/1 -> cram16/1(In1)
  "[17-17]"/1 -> uncram17/1(In)
  uncram17/1(Out1) -> acc17/1
  acc17/1 -> cram17/1(In1)
  "[18-18]"/1 -> uncram18/1(In)
  uncram18/1(Out1) -> acc18/1
  acc18/1 -> cram18/1(In1)
  "[19-19]"/1 -> uncram19/1(In)
  uncram19/1(Out1) -> acc19/1
  acc19/1 -> cram19/1(In1)
  "[20-20]"/1 -> uncram20/1(In)
  uncram20/1(Out1) -> acc20/1
  acc20/1 -> cram20/1(In1)
  "[21-21]"/1 -> uncram21/1(In)
  uncram21/1(Out1) -> acc21/1
  acc21/1 -> cram21/1(In1)
  "[22-22]"/1 -> uncram22/1(In)
  uncram22/1(Out1) -> acc22/1
  acc22/1 -> cram22/1(In1)
  "[23-23]"/1 -> uncram23/1(In)
  uncram23/1(Out1) -> acc23/1
  acc23/1 -> cram23/1(In1)
  "[24-24]"/1 -> uncram24/1(In)
  uncram24/1(Out1) -> acc24/1
  acc24/1 -> cram24/1(In1)
  "[25-25]"/1 -> uncram25/1(In)
  uncram25/1(Out1) -> acc25/1
  acc25/1 -> cram25/1(In1)
  "[26-26]"/1 -> uncram26/1(In)
  uncram26/1(Out1) -> acc26/1
  acc26/1 -> cram26/1(In1)
  "[27-27]"/1 -> uncram27/1(In)
  uncram27/1(Out1) -> acc27/1
  acc27/1 -> cram27/1(In1)
  "[28-28]"/1 -> uncram28/1(In)
  uncram28/1(Out1) -> acc28/1
  acc28/1 -> cram28/1(In1)
  "[29-29]"/1 -> uncram29/1(In)
  uncram29/1(Out1) -> acc29/1
  acc29/1 -> cram29/1(In1)
  "[30-30]"/1 -> uncram30/1(In)
  uncram30/1(Out1) -> acc30/1
  acc30/1 -> cram30/1(In1)
  "[31-31]"/1 -> uncram31/1(In)
  uncram31/1(Out1) -> acc31/1
  acc31/1 -> cram31/1(In1)
  acc0/3 -> stream_count/1, sync_out/1
  stream_count/1 -> mux/1
  cram0/1(Out) -> mux/2
  cram1/1(Out) -> mux/3
  cram2/1(Out) -> mux/4
  cram3/1(Out) -> mux/5
  cram4/1(Out) -> mux/6
  cram5/1(Out) -> mux/7
  cram6/1(Out) -> mux/8
  cram7/1(Out) -> mux/9
  cram8/1(Out) -> mux/10
  cram9/1(Out) -> mux/11
  cram10/1(Out) -> mux/12
  cram11/1(Out) -> mux/13
  cram12/1(Out) -> mux/14
  cram13/1(Out) -> mux/15
  cram14/1(Out) -> mux/16
  cram15/1(Out) -> mux/17
  cram16/1(Out) -> mux/18
  cram17/1(Out) -> mux/19
  cram18/1(Out) -> mux/20
  cram19/1(Out) -> mux/21
  cram20/1(Out) -> mux/22
  cram21/1(Out) -> mux/23
  cram22/1(Out) -> mux/24
  cram23/1(Out) -> mux/25
  cram24/1(Out) -> mux/26
  cram25/1(Out) -> mux/27
  cram26/1(Out) -> mux/28
  cram27/1(Out) -> mux/29
  cram28/1(Out) -> mux/30
  cram29/1(Out) -> mux/31
  cram30/1(Out) -> mux/32
  cram31/1(Out) -> mux/33
  mux/1 -> last_uncram/1(In)
  acc0/2 -> valid/1
  last_uncram/1(Out1) -> conv0/1
  conv0/1 -> "[n+0]"/1
